simulink model "controladorBH_ModeloHidraulico"  (R2022b)
settings: Solver=ode23s  StartTime=0.0  StopTime=5  FixedStep=1e-1  RelTol=1e-4
values from neighbouring files (symbols this model uses):
  A1 = 1.2566*10^-3    (= 0.0012566)    [BH_ModeloHidraulico.m]
  A2 = 8.7650*10^-4    (= 0.0008765)    [BH_ModeloHidraulico.m]
  Be = 9000*10^5    (= 900000000)    [BH_ModeloHidraulico.m]
  f = 1500    [BH_ModeloHidraulico.m]
  kc1 = 3.644*10^-12    (= 3.644e-12)    [BH_ModeloHidraulico.m]
  kc2 = 4.376*10^-12    (= 4.376e-12)    [BH_ModeloHidraulico.m]
  kq1 = 4.76*10^-4    (= 0.000476)    [BH_ModeloHidraulico.m]
  kq2 = 4.76*10^-4    (= 0.000476)    [BH_ModeloHidraulico.m]
  M = 84    [BH_ModeloHidraulico.m]
  V1 = Vl1+A1*xe0    (= 0.0001330412)    [BH_ModeloHidraulico.m]
  V2 = Vl2+A2*(L-xe0)    (= 0.000153427)    [BH_ModeloHidraulico.m]
undefined symbols (not defined in the file or in its folder): k
settings Model: Creator=beatr  LastModifiedBy=dsilva
settings DataIOCC: ReturnWorkspaceOutputs=off
settings DebuggingCC: UnconnectedInputMsg=warning  UnconnectedOutputMsg=warning  UnconnectedLineMsg=warning
settings ModelReferenceCC: EnableRefExpFcnMdlSchedulingChecks=on
settings RTWCC: DLArmComputeVersion=19.05

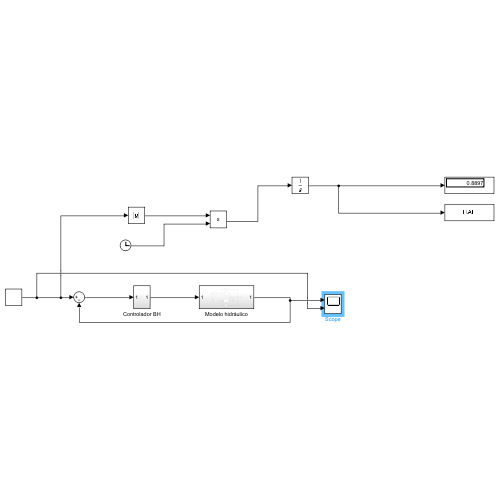
[thumbnail: Simulink's stored preview of the top-level diagram]
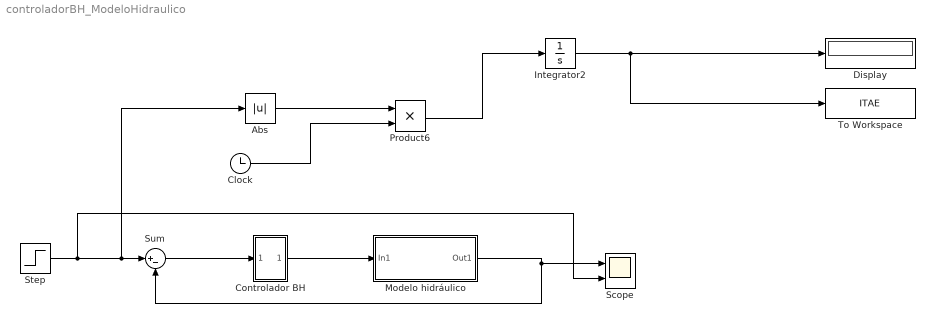
== system controladorBH_ModeloHidraulico ==
  Abs : Abs  SaturateOnIntegerOverflow=off
  Clock : Clock
  Controlador BH : Subsystem
  Display : Display
  Integrator2 : Integrator
  Modelo hidráulico : Subsystem
  Product6 : Product
  Scope : Scope  NumInputPorts=2
  Step : Step  SampleTime=0
  Sum : Sum  Inputs=|+-
  To Workspace : ToWorkspace  VariableName=ITAE  SampleTime=-1
  wires:
  Step/1 -> Scope/2, Abs/1, Sum/1
  Modelo hidráulico/1(Out1) -> Sum/2, Scope/1
  Controlador BH/1(Out1) -> Modelo hidráulico/1(In1)
  Sum/1 -> Controlador BH/1(In1)
  Integrator2/1 -> To Workspace/1, Display/1
  Product6/1 -> Integrator2/1
  Abs/1 -> Product6/1
  Clock/1 -> Product6/2

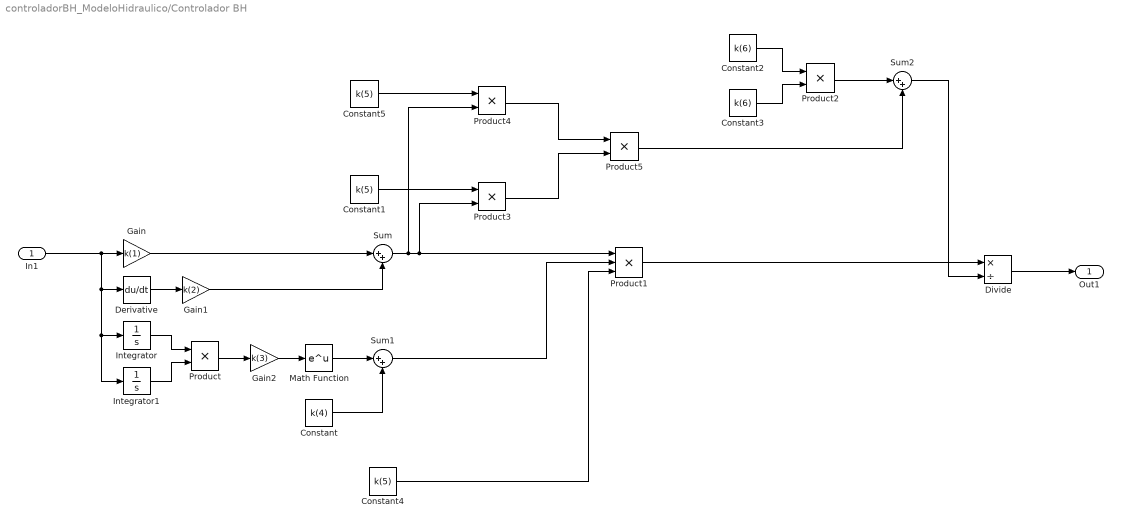
== system controladorBH_ModeloHidraulico/Controlador BH ==
  In1 : Inport
  Constant : Constant  Value=k(4)
  Constant1 : Constant  Value=k(5)
  Constant2 : Constant  Value=k(6)
  Constant3 : Constant  Value=k(6)
  Constant4 : Constant  Value=k(5)
  Constant5 : Constant  Value=k(5)
  Derivative : Derivative
  Divide : Product  Inputs=*/
  Gain : Gain  Gain=k(1)
  Gain1 : Gain  Gain=k(2)
  Gain2 : Gain  Gain=k(3)
  Integrator : Integrator
  Integrator1 : Integrator
  Math Function : Math
  Product{,2..5} (5 alike) : Product
  Product1 : Product  Inputs=3
  Sum : Sum  Inputs=|++
  Sum1 : Sum  Inputs=|++
  Sum2 : Sum  Inputs=|++
  Out1 : Outport
  wires:
  Derivative/1 -> Gain1/1
  Gain/1 -> Sum/1
  Gain1/1 -> Sum/2
  Integrator/1 -> Product/1
  Integrator1/1 -> Product/2
  Product/1 -> Gain2/1
  Gain2/1 -> Math Function/1
  Math Function/1 -> Sum1/1
  Constant/1 -> Sum1/2
  Product1/1 -> Divide/1
  Constant3/1 -> Product2/2
  Product2/1 -> Sum2/1
  Sum/1 -> Product4/2, Product3/2, Product1/1
  Sum1/1 -> Product1/2
  Constant4/1 -> Product1/3
  Constant1/1 -> Product3/1
  Constant5/1 -> Product4/1
  Product4/1 -> Product5/1
  Product3/1 -> Product5/2
  Product5/1 -> Sum2/2
  Sum2/1 -> Divide/2
  Divide/1 -> Out1/1
  In1/1 -> Integrator1/1, Integrator/1, Derivative/1, Gain/1
  Constant2/1 -> Product2/1

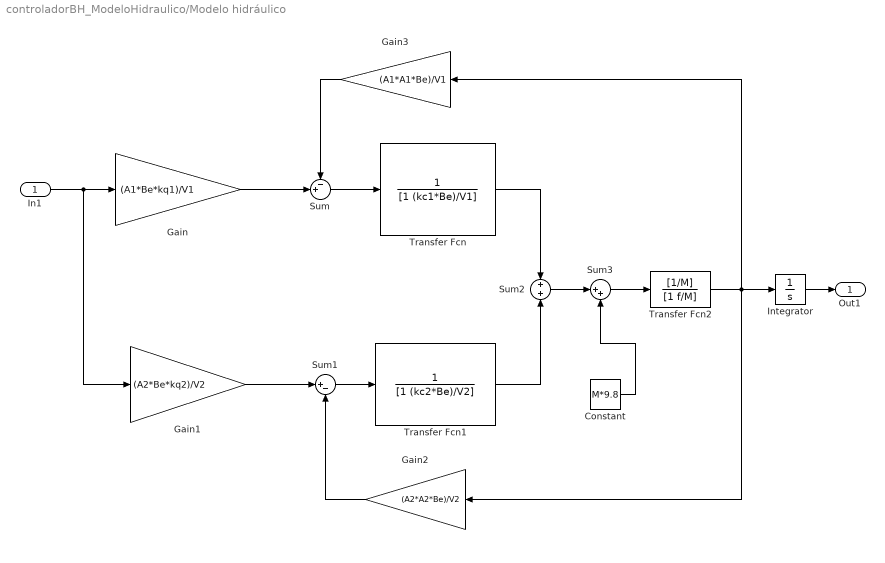
== system controladorBH_ModeloHidraulico/Modelo hidráulico ==
  In1 : Inport
  Constant : Constant  Value=M*9.8
  Gain : Gain  Gain=(A1*Be*kq1)/V1
  Gain1 : Gain  Gain=(A2*Be*kq2)/V2
  Gain2 : Gain  Gain=(A2*A2*Be)/V2
  Gain3 : Gain  Gain=(A1*A1*Be)/V1
  Integrator : Integrator
  Sum : Sum  Inputs=-+|
  Sum1 : Sum  Inputs=|+-
  Sum2 : Sum  Inputs=+|+
  Sum3 : Sum  Inputs=|++
  Transfer Fcn : TransferFcn  Denominator=[1 (kc1*Be)/V1]
  Transfer Fcn1 : TransferFcn  Denominator=[1 (kc2*Be)/V2]
  Transfer Fcn2 : TransferFcn  Numerator=[1/M]  Denominator=[1 f/M]
  Out1 : Outport
  wires:
  Constant/1 -> Sum3/2
  Sum2/1 -> Sum3/1
  Sum3/1 -> Transfer Fcn2/1
  Transfer Fcn2/1 -> Integrator/1, Gain3/1, Gain2/1
  Gain3/1 -> Sum/1
  In1/1 -> Gain1/1, Gain/1
  Gain1/1 -> Sum1/1
  Transfer Fcn1/1 -> Sum2/2
  Sum1/1 -> Transfer Fcn1/1
  Gain2/1 -> Sum1/2
  Sum/1 -> Transfer Fcn/1
  Transfer Fcn/1 -> Sum2/1
  Integrator/1 -> Out1/1
  Gain/1 -> Sum/2
